simulink model "Laengsdynamikmodell_NEmo_MonteCarlo"  (R2019b)
settings: Solver=FixedStepAuto  StartTime=0.0  StopTime=1  FixedStep=SampleTime  RelTol=1e-3
undefined symbols (not defined in the file): C_RR, DiscIntNeverNeededParam, gravity, OM_PEl_M_Map, omega_Mot, PEl_MotVector, power_map_Mot, r_dyn, torque_Mot, UncertaintyMappedLosses, UncertaintyRollerDynamometer, UncertaintyTabledConsumption, VehMass
libraries: Driver_PI x1, Longitudinal_DrivingCycles x1, Acceleration_Calculation x1, Air_Resistance x1, Roll_Resistance x1, Slope_Resistance x1, Simple_Auxiliary x1, Gear_Stage x1, DCAC_Converter x1
(part 2 of 2)

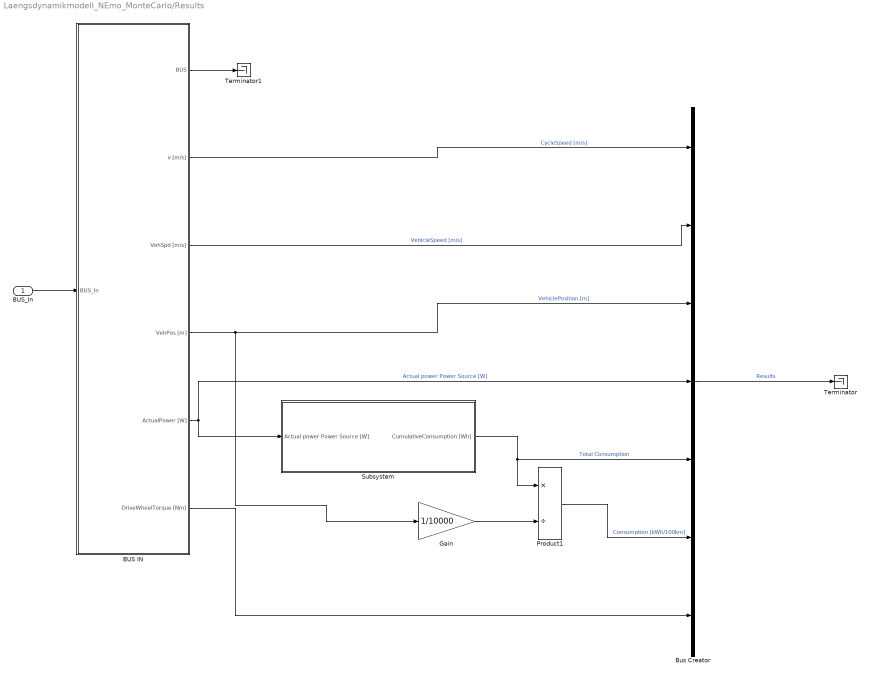
== system Laengsdynamikmodell_NEmo_MonteCarlo/Results ==
  BUS_In : Inport
  BUS IN : Subsystem
      mask help:
      | <Author> Alexander Koch
      | <Date> 02/05/2017
      | <Predecessor> Stefan Müller, Stephan Rohr
      |
      | <Description>
      | Automated BUS IN Block for the Bus System. After the Bus In is connected and receives signals it is possible to choose the required signals by clicking on the block. After choosing the signals it is possible to push the Refresh button. This button builds the required amount of outputs, connects the Bus Selector and the Outputs and rename all the outputs with the corresponding signal name.
      |
      | The Block automaticlly disconnects the link to the library block after opening the first time
      |
      | <Parameters>
      | -
      |
      | <Inputs>
      | Bus [Bus]
      |
      | <Outputs>
      | Bus [Bus]
      | SignalName[-]
      mask init:
      | BusInInitFct()
      settings: OpenFcn=|
      | set_param(gcb(),'LinkStatus','none')
      | open_system(gcb(),'mask')
      | open_system(strcat(gcb(),'/Bus Selector'),'Parameter')
      mask DialogControl ParameterGroupVar Prompt: Refresh
      mask DialogControl RefreshOutputs Prompt: Refresh all Output Names
      mask DialogControl RefreshOutputs Callback: BusInInitFct()
  Bus Creator : BusCreator  Inputs=7
  Gain : Gain  Gain=1/10000
  Product1 : Product  Inputs=*/
  Subsystem : Subsystem
  Terminator : Terminator
  Terminator1 : Terminator
  wires:
  BUS_In/1 -> BUS IN/1(BUS_In)
  BUS IN/1(BUS) -> Terminator1/1
  Bus Creator/1 -> Terminator/1  "Results"
  BUS IN/5(ActualPower [W]) -> Bus Creator/4, Subsystem/1(Actual power Power Source [W])  "Actual power Power Source [W]"
  BUS IN/2(v [m/s]) -> Bus Creator/1  "CycleSpeed [m/s]"
  BUS IN/3(VehSpd [m/s]) -> Bus Creator/2  "VehicleSpeed [m/s]"
  BUS IN/4(VehPos [m]) -> Bus Creator/3, Gain/1  "VehiclePosition [m]"
  BUS IN/6(DriveWheelTorque [Nm]) -> Bus Creator/7
  Gain/1 -> Product1/2
  Product1/1 -> Bus Creator/6  "Consumption [kWh/100km]"
  Subsystem/1(CumulativeConsumption [Wh]) -> Bus Creator/5, Product1/1  "Total Consumption"

== system Laengsdynamikmodell_NEmo_MonteCarlo/Timer and Bus Reset ==
  BUS_In : Inport
  Bus Creator : BusCreator  Inputs=1
  Bus Selector : BusSelector  OutputSignals=Dynamics,Powertrain,Powersource,VehicleControlUnit,Driver and Enironment,DrivinCycle  OutputAsBus=on
  Unit Delay : UnitDelay  SampleTime=-1  HasFrameUpgradeWarning=on
  BUS_Out : Outport  VectorParamsAs1DForOutWhenUnconnected=off
  wires:
  Bus Creator/1 -> BUS_Out/1
  Bus Selector/1 -> Unit Delay/1
  Unit Delay/1 -> Bus Creator/1  "Bus_Old"
  BUS_In/1 -> Bus Selector/1

== system Laengsdynamikmodell_NEmo_MonteCarlo/Vehicle Control Unit ==
  BUS_In : Inport
  BUS IN : Subsystem
      mask help:
      | <Author> Alexander Koch based on Stefan Müller, Stephan Rohr
      | <Date> 02/05/2017
      |
      | <Description>
      | Automated BUS IN Block for the Bus System. After the Bus In is connected and receives signals it is possible to choose the required signals by clicking on the block. After choosing the signals it is possible to push the Refresh button. This button builds the required amount of outputs, connects the Bus Selector and the Outputs and rename all the outputs with the corresponding signal name.
      |
      | The Block automaticlly disconnects the link to the library block after opening the first time
      |
      | <Parameters>
      | -
      |
      | <Inputs>
      | Bus [Bus]
      |
      | <Outputs>
      | Bus [Bus]
      | SignalName[-]
      mask init:
      | BusInInitFct()
      settings: OpenFcn=|
      | set_param(gcb(),'LinkStatus','none')
      | open_system(gcb(),'mask')
      | open_system(strcat(gcb(),'/Bus Selector'),'Parameter')
      mask DialogControl ParameterGroupVar Prompt: Refresh
      mask DialogControl RefreshOutputs Prompt: Refresh all Output Names
      mask DialogControl RefreshOutputs Callback: BusInInitFct()
  BUS OUT : Subsystem  mask{NumberofInputs=3, NameSys='VehicleControlUnit'}
      mask prompts: NumberofInputs "Numper of costum inputs"; NameSys "Name of Bus Subsystem"
      mask help:
      | <Author> Alexander Koch based on Stefan Müller, Stephan Rohr
      | <Date> 02/05/2017
      |
      | <Description>
      | Automated BUS Out Block for the Bus System. Allows to enter the Number of costum inputs and the name of the bus system. After entering the parameters the required amout of Inputs are built and connected to the Bus Creator. The signal names that are connected to the inputs In1, ..., InN are automatically adopted at the Bus signal names and can be found in the Bus under the name of the Bus Subsystem. If the signal (line) to the Inport has no name, the name of the previous blocks outport is taken. If this is not possible, the name if the previous block is taken for the Bus signal name.
      |
      | Additional, there are two buttons. The Refresh Input Names refreshes all Input Names. This is required if signal names are changed or signals are connected for the first time. To build a new system or if another Subsystem is added between existing subsystems, the Refresh Bus Selector is required at every subsystem that is calculated after the new subsystem.
      |
      | The Block automaticlly disconnects the link to the library block after opening the first time
      |
      | <Parameters>
      | Number of costum inputs [-]
      | Name of Bus Subsystem ['abc']
      |
      | <Inputs>
      | Bus [Bus]
      | In1 [ ]
      |
      | <Outputs>
      | Bus [Bus]
      mask init:
      | BusRefreshInputs()
      settings: OpenFcn=|
      | set_param(gcb(),'LinkStatus','none')
      | open_system(gcb(),'mask')
      mask DialogControl Container3 Prompt: Refresh
      mask DialogControl RefreshInputNames Prompt: Refresh Input Names
      mask DialogControl RefreshInputNames Callback: BusRefreshLineNames()
      mask DialogControl RefreshBusSelector Prompt: Refresh Bus Selector
      mask DialogControl RefreshBusSelector Callback: BusRefreshBusSelector()
  Control Unit Simple : Subsystem  AncestorBlock=Control_Unit_Simple/Control Unit Simple  mask(SB){Brake_Distribution_Front=0.7, MaxBrkTrq=448, MaxMotorTrq=110}
      mask prompts: Brake_Distribution_Front "Brake Distribution Front"; MaxBrkTrq "Maximal Braking Torque"; MaxMotorTrq "Maximal Motor Torque"
      mask help:
      | <Author> Alexander Koch based on Stefan Müller, Stephan Rohr </Author>
      | <Date> 03/04/2017 </Date>
      |
      | <Description>
      | Requires acceleration pedal position, braking pedal position, a brake distribution, the maximal possible braking torque and tha maximal motor torque and calculates a target drive system torque and a target braking torque for front and rear axle. Minimum drive torques is zero.
      | </Description>
      mask Help:
      | <Parameters>
      | Brake distribution front [-]
      | 	<Min> 0 </Min>
      | 	<Max> 1 </Max>
      | Maximal braking torque [Nm]
      | Maximal motor torque [Nm]
      | </Parameters>
      | 
      | <Inputs>
      | AccPedalPos [-]
      | 	<Min> 0 </Min>
      | 	<Max> 1 </Max>
      | BrakePedalPos [-]
      | 	<Min>0 </Min>
      | 	<Max> 1 </Max>
      | </Inputs>
      | 
      | <Outputs>
      | TargetDriveTrq [Nm]
      | 	<Min> 0 </Min>
      | TargetBrakeTrqFrontAxle [Nm]
      | 	<Max> 0 </Max>
      | TargetBrakeTrqRearAxle [Nm]
      | 	<Max> 0 </Max>
      | </Outputs>
      mask TypeOptions Brake_Distribution_Front: Brake_Distribution_Front/Value
      mask TypeOptions MaxBrkTrq: MaxBrakeTorque/Value
      mask TypeOptions MaxMotorTrq: MaxMotorTorque/Value
      mask DialogControl Container3 Prompt: Documentation:
      mask DialogControl DescHelpVar Prompt: %<MaskHelp>
  BUS_Out : Outport  VectorParamsAs1DForOutWhenUnconnected=off
  wires:
  BUS IN/1(BUS) -> BUS OUT/1(BUS)
  BUS OUT/1(BUS_OUT) -> BUS_Out/1
  BUS_In/1 -> BUS IN/1(BUS_In)
  Control Unit Simple/2(TargetBrakeTrqFrontAxle [Nm]) -> BUS OUT/3(In2)
  Control Unit Simple/3(TargetBrakeTrqRearAxle [Nm]) -> BUS OUT/4(In3)
  Control Unit Simple/1("TargetDriveTrq [Nm] ") -> BUS OUT/2(In1)
  BUS IN/2(AccPedalPos [-]) -> Control Unit Simple/1(AccPedalPos [-])
  BUS IN/3(BrakePedalPos [-]) -> Control Unit Simple/2(BrakePedalPos [-])

== system Laengsdynamikmodell_NEmo_MonteCarlo/Driver and Environment/BUS IN ==
  BUS_In : Inport
  Bus Selector : BusSelector  OutputSignals=DrivinCycle.v [m/s],Bus_Old.Dynamics.VehSpd [m/s]
  BUS : Outport  VectorParamsAs1DForOutWhenUnconnected=off
  v [m/s] : Outport  Port=2  VectorParamsAs1DForOutWhenUnconnected=off
  VehSpd [m/s] : Outport  Port=3  VectorParamsAs1DForOutWhenUnconnected=off
  wires:
  BUS_In/1 -> Bus Selector/1, BUS/1
  Bus Selector/1 -> v [m/s]/1  "<v [m/s]>"
  Bus Selector/2 -> VehSpd [m/s]/1  "<VehSpd [m/s]>"

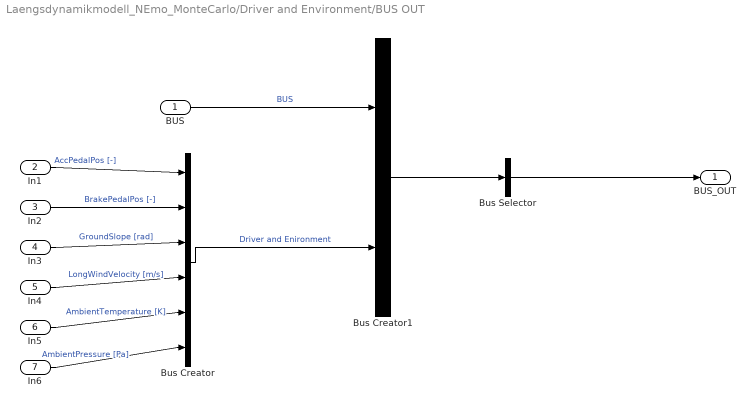
== system Laengsdynamikmodell_NEmo_MonteCarlo/Driver and Environment/BUS OUT ==
  BUS : Inport
  In1 : Inport  Port=2
  In2 : Inport  Port=3
  In3 : Inport  Port=4
  In4 : Inport  Port=5
  In5 : Inport  Port=6
  In6 : Inport  Port=7
  Bus Creator : BusCreator  Inputs=NumberofInputs
  Bus Creator1 : BusCreator  Inputs=2
  Bus Selector : BusSelector  OutputSignals=Driver and Enironment,BUS.DrivinCycle,BUS.Bus_Old  OutputAsBus=on
  BUS_OUT : Outport  VectorParamsAs1DForOutWhenUnconnected=off
  wires:
  Bus Creator1/1 -> Bus Selector/1
  BUS/1 -> Bus Creator1/1  "BUS"
  Bus Creator/1 -> Bus Creator1/2  "Driver and Enironment"
  Bus Selector/1 -> BUS_OUT/1
  In1/1 -> Bus Creator/1  "AccPedalPos [-]"
  In2/1 -> Bus Creator/2  "BrakePedalPos [-]"
  In3/1 -> Bus Creator/3  "GroundSlope [rad]"
  In4/1 -> Bus Creator/4  "LongWindVelocity [m/s]"
  In5/1 -> Bus Creator/5  "AmbientTemperature [K]"
  In6/1 -> Bus Creator/6  "AmbientPressure [Pa]"

== system Laengsdynamikmodell_NEmo_MonteCarlo/Driver and Environment/Constant Environment ==
  Const_Ambient_Pressure : Constant  Value=Ambient_P  SampleTime=LocalSampleTime
  Const_Ambient_Temperature : Constant  Value=Ambient_Temp  SampleTime=LocalSampleTime
  Const_Ground_Slope : Constant  Value=Ground_Slope  SampleTime=LocalSampleTime
  Const_Long_Wind_Velocity : Constant  Value=Long_Wind_Speed  SampleTime=LocalSampleTime
  GroundSlope [rad] : Outport  SampleTime=GlobalSampleTime  VectorParamsAs1DForOutWhenUnconnected=off
  LongWindVelocity [m/s] : Outport  Port=2  SampleTime=GlobalSampleTime  VectorParamsAs1DForOutWhenUnconnected=off
  AmbientTemperature [K] : Outport  Port=3  SampleTime=GlobalSampleTime  VectorParamsAs1DForOutWhenUnconnected=off
  AmbientPressure [Pa] : Outport  Port=4  SampleTime=GlobalSampleTime  VectorParamsAs1DForOutWhenUnconnected=off
  wires:
  Const_Ambient_Pressure/1 -> AmbientPressure [Pa]/1
  Const_Ambient_Temperature/1 -> AmbientTemperature [K]/1
  Const_Ground_Slope/1 -> GroundSlope [rad]/1
  Const_Long_Wind_Velocity/1 -> LongWindVelocity [m/s]/1

== system Laengsdynamikmodell_NEmo_MonteCarlo/Driving Cycle/BUS IN ==
  BUS_In : Inport
  Bus Selector : BusSelector  OutputSignals=Bus_Old.Dynamics.VehSpd [m/s]
  BUS : Outport  VectorParamsAs1DForOutWhenUnconnected=off
  VehSpd [m/s] : Outport  Port=2  VectorParamsAs1DForOutWhenUnconnected=off
  wires:
  BUS_In/1 -> Bus Selector/1, BUS/1
  Bus Selector/1 -> VehSpd [m/s]/1  "<VehSpd [m/s]>"

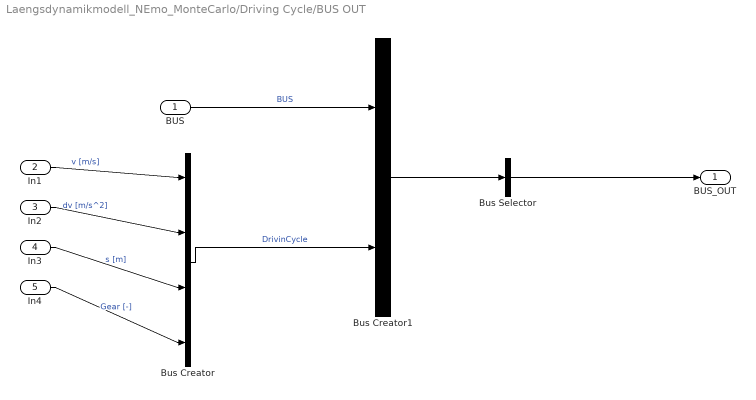
== system Laengsdynamikmodell_NEmo_MonteCarlo/Driving Cycle/BUS OUT ==
  BUS : Inport
  In1 : Inport  Port=2
  In2 : Inport  Port=3
  In3 : Inport  Port=4
  In4 : Inport  Port=5
  Bus Creator : BusCreator  Inputs=NumberofInputs
  Bus Creator1 : BusCreator  Inputs=2
  Bus Selector : BusSelector  OutputSignals=DrivinCycle,BUS.Bus_Old  OutputAsBus=on
  BUS_OUT : Outport  VectorParamsAs1DForOutWhenUnconnected=off
  wires:
  Bus Creator1/1 -> Bus Selector/1
  BUS/1 -> Bus Creator1/1  "BUS"
  Bus Creator/1 -> Bus Creator1/2  "DrivinCycle"
  Bus Selector/1 -> BUS_OUT/1
  In1/1 -> Bus Creator/1  "v [m/s]"
  In2/1 -> Bus Creator/2  "dv [m/s^2]"
  In3/1 -> Bus Creator/3  "s [m]"
  In4/1 -> Bus Creator/4  "Gear [-]"

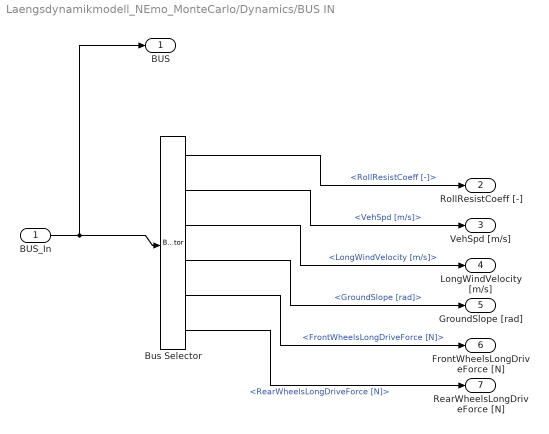
== system Laengsdynamikmodell_NEmo_MonteCarlo/Dynamics/BUS IN ==
  BUS_In : Inport
  Bus Selector : BusSelector  OutputSignals=Powertrain.RollResistCoeff [-],Bus_Old.Dynamics.VehSpd [m/s],Driver and Enironment.LongWindVelocity [m/s],Driver and Enironment.GroundSlope [rad],Powertrain.FrontWheelsLongDriveForce [N],Powertrain.RearWheelsLongDriveForce [N]
  BUS : Outport  VectorParamsAs1DForOutWhenUnconnected=off
  RollResistCoeff [-] : Outport  Port=2  VectorParamsAs1DForOutWhenUnconnected=off
  VehSpd [m/s] : Outport  Port=3  VectorParamsAs1DForOutWhenUnconnected=off
  LongWindVelocity [m/s] : Outport  Port=4  VectorParamsAs1DForOutWhenUnconnected=off
  GroundSlope [rad] : Outport  Port=5  VectorParamsAs1DForOutWhenUnconnected=off
  FrontWheelsLongDriveForce [N] : Outport  Port=6  VectorParamsAs1DForOutWhenUnconnected=off
  RearWheelsLongDriveForce [N] : Outport  Port=7  VectorParamsAs1DForOutWhenUnconnected=off
  wires:
  BUS_In/1 -> Bus Selector/1, BUS/1
  Bus Selector/1 -> RollResistCoeff [-]/1  "<RollResistCoeff [-]>"
  Bus Selector/2 -> VehSpd [m/s]/1  "<VehSpd [m/s]>"
  Bus Selector/3 -> LongWindVelocity [m/s]/1  "<LongWindVelocity [m/s]>"
  Bus Selector/4 -> GroundSlope [rad]/1  "<GroundSlope [rad]>"
  Bus Selector/5 -> FrontWheelsLongDriveForce [N]/1  "<FrontWheelsLongDriveForce [N]>"
  Bus Selector/6 -> RearWheelsLongDriveForce [N]/1  "<RearWheelsLongDriveForce [N]>"

== system Laengsdynamikmodell_NEmo_MonteCarlo/Dynamics/BUS OUT ==
  BUS : Inport
  In1 : Inport  Port=2
  In2 : Inport  Port=3
  In3 : Inport  Port=4
  Bus Creator : BusCreator  Inputs=NumberofInputs
  Bus Creator1 : BusCreator  Inputs=2
  Bus Selector : BusSelector  OutputSignals=Dynamics,BUS.Powertrain,BUS.Powersource,BUS.VehicleControlUnit,BUS.Driver and Enironment,BUS.DrivinCycle,BUS.Bus_Old  OutputAsBus=on
  BUS_OUT : Outport  VectorParamsAs1DForOutWhenUnconnected=off
  wires:
  Bus Creator1/1 -> Bus Selector/1
  BUS/1 -> Bus Creator1/1  "BUS"
  Bus Creator/1 -> Bus Creator1/2  "Dynamics"
  Bus Selector/1 -> BUS_OUT/1
  In1/1 -> Bus Creator/1  "Acc [m/s^2]"
  In2/1 -> Bus Creator/2  "VehSpd [m/s]"
  In3/1 -> Bus Creator/3  "VehPos [m]"

== system Laengsdynamikmodell_NEmo_MonteCarlo/Power Source/BUS IN ==
  BUS_In : Inport
  Bus Selector : BusSelector  OutputSignals=Bus_Old.Powertrain.PowertrainPowerReq [W]
  BUS : Outport  VectorParamsAs1DForOutWhenUnconnected=off
  PowertrainPowerReq [W] : Outport  Port=2  VectorParamsAs1DForOutWhenUnconnected=off
  wires:
  BUS_In/1 -> Bus Selector/1, BUS/1
  Bus Selector/1 -> PowertrainPowerReq [W]/1  "<PowertrainPowerReq [W]>"

== system Laengsdynamikmodell_NEmo_MonteCarlo/Power Source/BUS OUT ==
  BUS : Inport
  In1 : Inport  Port=2
  In2 : Inport  Port=3
  In3 : Inport  Port=4
  Bus Creator : BusCreator  Inputs=NumberofInputs
  Bus Creator1 : BusCreator  Inputs=2
  Bus Selector : BusSelector  OutputSignals=Powersource,BUS.VehicleControlUnit,BUS.Driver and Enironment,BUS.DrivinCycle,BUS.Bus_Old  OutputAsBus=on
  BUS_OUT : Outport  VectorParamsAs1DForOutWhenUnconnected=off
  wires:
  Bus Creator1/1 -> Bus Selector/1
  BUS/1 -> Bus Creator1/1  "BUS"
  Bus Creator/1 -> Bus Creator1/2  "Powersource"
  Bus Selector/1 -> BUS_OUT/1
  In1/1 -> Bus Creator/1  "ActualPower [W]"
  In2/1 -> Bus Creator/2  "MaxPower [W]"
  In3/1 -> Bus Creator/3  "MinPower [W]"

== system Laengsdynamikmodell_NEmo_MonteCarlo/Power Source/Constant Power Source ==
  RequiredPower [W] : Inport
  Constant : Constant  Value=MaxPower
  Constant1 : Constant  Value=MinPower
  Saturation : Saturate  UpperLimit=MaxPower  LowerLimit=MinPower
  ActualPower [W] : Outport  VectorParamsAs1DForOutWhenUnconnected=off
  MaxPower [W] : Outport  Port=2  VectorParamsAs1DForOutWhenUnconnected=off
  MinPower [W] : Outport  Port=3  VectorParamsAs1DForOutWhenUnconnected=off
  wires:
  Constant/1 -> MaxPower [W]/1
  Constant1/1 -> MinPower [W]/1
  Saturation/1 -> ActualPower [W]/1
  RequiredPower [W]/1 -> Saturation/1

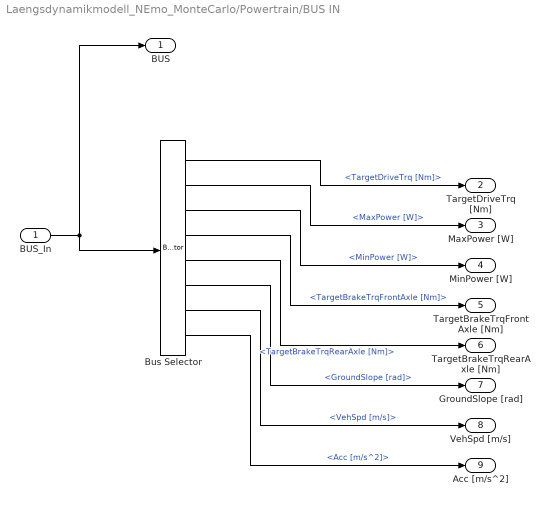
== system Laengsdynamikmodell_NEmo_MonteCarlo/Powertrain/BUS IN ==
  BUS_In : Inport
  Bus Selector : BusSelector  OutputSignals=VehicleControlUnit.TargetDriveTrq [Nm],Powersource.MaxPower [W],Powersource.MinPower [W],VehicleControlUnit.TargetBrakeTrqFrontAxle [Nm],VehicleControlUnit.TargetBrakeTrqRearAxle [Nm],Driver and Enironment.GroundSlope [rad],Bus_Old.Dynamics.VehSpd [m/s],Bus_Old.Dynamics.Acc [m/s^2]
  BUS : Outport  VectorParamsAs1DForOutWhenUnconnected=off
  TargetDriveTrq [Nm] : Outport  Port=2  VectorParamsAs1DForOutWhenUnconnected=off
  MaxPower [W] : Outport  Port=3  VectorParamsAs1DForOutWhenUnconnected=off
  MinPower [W] : Outport  Port=4  VectorParamsAs1DForOutWhenUnconnected=off
  TargetBrakeTrqFrontAxle [Nm] : Outport  Port=5  VectorParamsAs1DForOutWhenUnconnected=off
  TargetBrakeTrqRearAxle [Nm] : Outport  Port=6  VectorParamsAs1DForOutWhenUnconnected=off
  GroundSlope [rad] : Outport  Port=7  VectorParamsAs1DForOutWhenUnconnected=off
  VehSpd [m/s] : Outport  Port=8  VectorParamsAs1DForOutWhenUnconnected=off
  Acc [m/s^2] : Outport  Port=9  VectorParamsAs1DForOutWhenUnconnected=off
  wires:
  BUS_In/1 -> Bus Selector/1, BUS/1
  Bus Selector/1 -> TargetDriveTrq [Nm]/1  "<TargetDriveTrq [Nm]>"
  Bus Selector/2 -> MaxPower [W]/1  "<MaxPower [W]>"
  Bus Selector/3 -> MinPower [W]/1  "<MinPower [W]>"
  Bus Selector/4 -> TargetBrakeTrqFrontAxle [Nm]/1  "<TargetBrakeTrqFrontAxle [Nm]>"
  Bus Selector/5 -> TargetBrakeTrqRearAxle [Nm]/1  "<TargetBrakeTrqRearAxle [Nm]>"
  Bus Selector/6 -> GroundSlope [rad]/1  "<GroundSlope [rad]>"
  Bus Selector/7 -> VehSpd [m/s]/1  "<VehSpd [m/s]>"
  Bus Selector/8 -> Acc [m/s^2]/1  "<Acc [m/s^2]>"

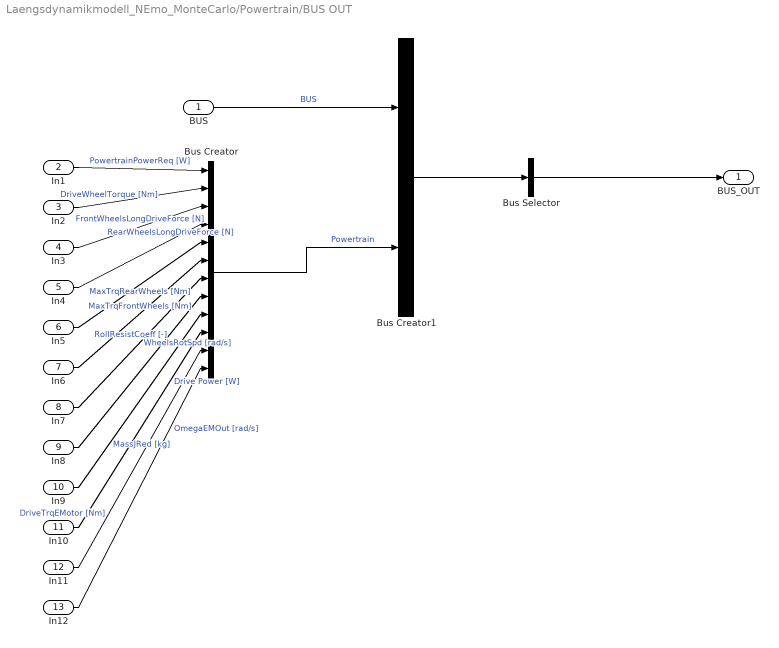
== system Laengsdynamikmodell_NEmo_MonteCarlo/Powertrain/BUS OUT ==
  BUS : Inport
  In1 : Inport  Port=2
  In2 : Inport  Port=3
  In3 : Inport  Port=4
  In4 : Inport  Port=5
  In5 : Inport  Port=6
  In6 : Inport  Port=7
  In7 : Inport  Port=8
  In8 : Inport  Port=9
  In9 : Inport  Port=10
  In10 : Inport  Port=11
  In11 : Inport  Port=12
  In12 : Inport  Port=13
  Bus Creator : BusCreator  Inputs=NumberofInputs
  Bus Creator1 : BusCreator  Inputs=2
  Bus Selector : BusSelector  OutputSignals=Powertrain,BUS.Powersource,BUS.VehicleControlUnit,BUS.Driver and Enironment,BUS.DrivinCycle,BUS.Bus_Old  OutputAsBus=on
  BUS_OUT : Outport  VectorParamsAs1DForOutWhenUnconnected=off
  wires:
  Bus Creator1/1 -> Bus Selector/1
  BUS/1 -> Bus Creator1/1  "BUS"
  Bus Creator/1 -> Bus Creator1/2  "Powertrain"
  Bus Selector/1 -> BUS_OUT/1
  In1/1 -> Bus Creator/1  "PowertrainPowerReq [W]"
  In2/1 -> Bus Creator/2  "DriveWheelTorque [Nm]"
  In3/1 -> Bus Creator/3  "FrontWheelsLongDriveForce [N]"
  In4/1 -> Bus Creator/4  "RearWheelsLongDriveForce [N]"
  In5/1 -> Bus Creator/5  "MaxTrqRearWheels [Nm]"
  In6/1 -> Bus Creator/6  "MaxTrqFrontWheels [Nm]"
  In7/1 -> Bus Creator/7  "WheelsRotSpd [rad/s]"
  In8/1 -> Bus Creator/8  "RollResistCoeff [-]"
  In9/1 -> Bus Creator/9  "MassJRed [kg]"
  In10/1 -> Bus Creator/10  "Drive Power [W]"
  In11/1 -> Bus Creator/11  "DriveTrqEMotor [Nm]"
  In12/1 -> Bus Creator/12  "OmegaEMOut [rad/s]"

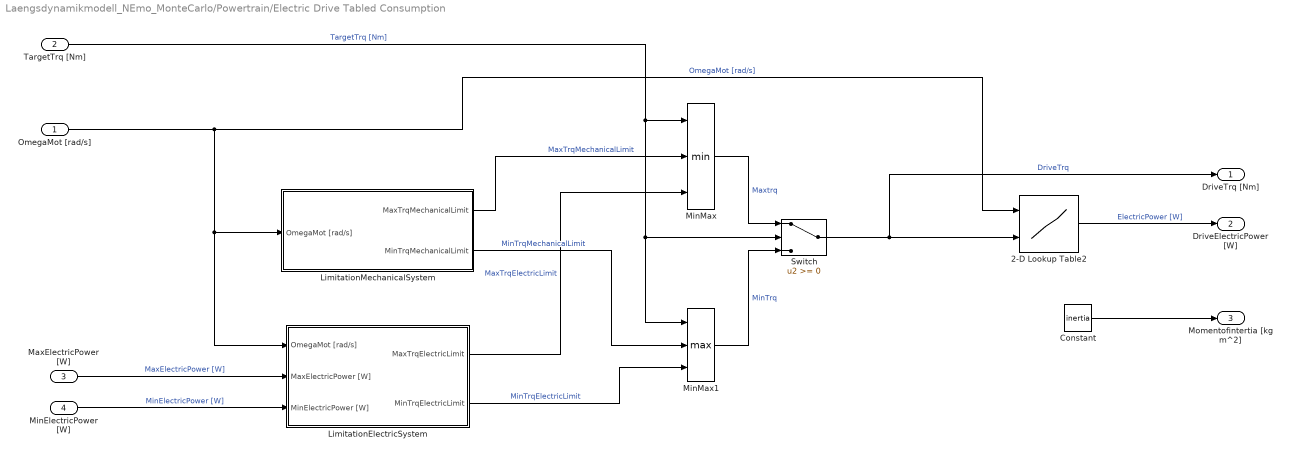
== system Laengsdynamikmodell_NEmo_MonteCarlo/Powertrain/Electric Drive Tabled Consumption ==
  OmegaMot [rad/s] : Inport  SampleTime=LocalSampleTime
  TargetTrq [Nm] : Inport  Port=2  SampleTime=LocalSampleTime
  MaxElectricPower [W] : Inport  Port=3  SampleTime=LocalSampleTime
  MinElectricPower [W] : Inport  Port=4  SampleTime=LocalSampleTime
  2-D Lookup Table2 : Lookup_n-D  BreakpointsForDimension1=OM_MotVector  BreakpointsForDimension2=M_MotVector  Table=OM_M_Pel_Map  UseLastTableValue=on  InternalRulePriority=Speed  RndMeth=Simplest  InputSameDT=on
  Constant : Constant  Value=inertia
  LimitationElectricSystem : Subsystem
  LimitationMechanicalSystem : Subsystem
  MinMax : MinMax  Inputs=3
  MinMax1 : MinMax  Function=max  Inputs=3
  Switch : Switch
  DriveTrq [Nm] : Outport  SampleTime=GlobalSampleTime  VectorParamsAs1DForOutWhenUnconnected=off
  DriveElectricPower [W] : Outport  Port=2  SampleTime=GlobalSampleTime  VectorParamsAs1DForOutWhenUnconnected=off
  Momentofintertia [kg m^2] : Outport  Port=3  SampleTime=GlobalSampleTime  VectorParamsAs1DForOutWhenUnconnected=off
  wires:
  Constant/1 -> Momentofintertia [kg m^2]/1
  LimitationElectricSystem/1(MaxTrqElectricLimit) -> MinMax/3  "MaxTrqElectricLimit"
  LimitationElectricSystem/2(MinTrqElectricLimit) -> MinMax1/3  "MinTrqElectricLimit"
  LimitationMechanicalSystem/2(MinTrqMechanicalLimit) -> MinMax1/2  "MinTrqMechanicalLimit"
  LimitationMechanicalSystem/1(MaxTrqMechanicalLimit) -> MinMax/2  "MaxTrqMechanicalLimit"
  MinElectricPower [W]/1 -> LimitationElectricSystem/3(MinElectricPower [W])  "MinElectricPower [W]"
  MaxElectricPower [W]/1 -> LimitationElectricSystem/2(MaxElectricPower [W])  "MaxElectricPower [W]"
  OmegaMot [rad/s]/1 -> 2-D Lookup Table2/1, LimitationMechanicalSystem/1(OmegaMot [rad/s]), LimitationElectricSystem/1(OmegaMot [rad/s])  "OmegaMot [rad/s]"
  Switch/1 -> DriveTrq [Nm]/1, 2-D Lookup Table2/2  "DriveTrq"
  TargetTrq [Nm]/1 -> MinMax/1, Switch/2, MinMax1/1  "TargetTrq [Nm]"
  MinMax1/1 -> Switch/3  "MinTrq"
  MinMax/1 -> Switch/1  "Maxtrq"
  2-D Lookup Table2/1 -> DriveElectricPower [W]/1  "ElectricPower [W]"

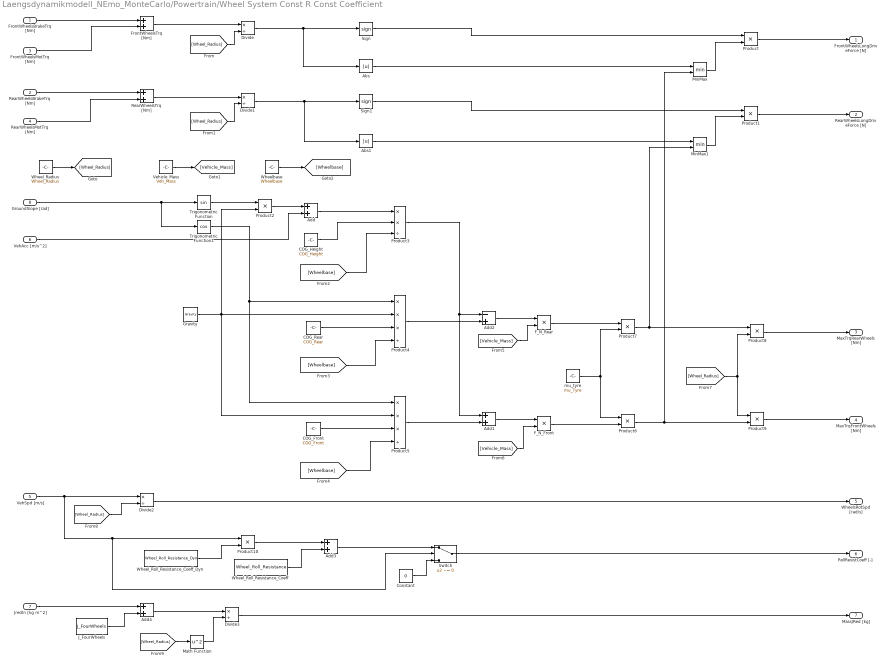
== system Laengsdynamikmodell_NEmo_MonteCarlo/Powertrain/Wheel System Const R Const Coefficient ==
  FrontWheelsBrakeTrq [Nm] : Inport  SampleTime=LocalSampleTime
  RearWheelsBrakeTrq [Nm] : Inport  Port=2  SampleTime=LocalSampleTime
  FrontWheelsMotTrq [Nm] : Inport  Port=3  SampleTime=LocalSampleTime
  RearWheelsMotTrq [Nm] : Inport  Port=4  SampleTime=LocalSampleTime
  VehSpd [m/s] : Inport  Port=5  SampleTime=LocalSampleTime
  VehAcc [m/s^2] : Inport  Port=6  SampleTime=LocalSampleTime
  JredIn [kg m^2] : Inport  Port=7  SampleTime=LocalSampleTime
  GroundSlope [rad] : Inport  Port=8  SampleTime=LocalSampleTime
  Abs : Abs
  Abs1 : Abs
  Add{,1,3..4} (4 alike) : Sum
  Add2 : Sum  Inputs=-+
  COG_Front : Constant  Value=COG_Front
  COG_Height : Constant  Value=COG_Height
  COG_Rear : Constant  Value=COG_Rear
  Constant : Constant  Value=0
  Divide{,1..3} (4 alike) : Product  Inputs=*/
  F_N_Front : Product
  F_N_Rear : Product
  FrontWheelsTrq [Nm] : Sum
  Gravity : Constant  Value=Gravity
  J_FourWheels : Constant  Value=J_FourWheels
  Math Function : Math  Operator=square  SaturateOnIntegerOverflow=on
  MinMax : MinMax  Inputs=2
  MinMax1 : MinMax  Inputs=2
  Product{,1..2,6..10} (8 alike) : Product
  Product3 : Product  Inputs=**/
  Product4 : Product  Inputs=***/
  Product5 : Product  Inputs=***/
  RearWheelsTrq [Nm] : Sum
  Sign : Signum
  Sign1 : Signum
  Switch : Switch  Criteria=u2 ~= 0
  Trigonometric Function : Trigonometry
  Trigonometric Function1 : Trigonometry  Operator=cos
  Vehicle_Mass : Constant  Value=Veh_Mass
  Wheel_Radius : Constant  Value=Wheel_Radius
  Wheel_Roll_Resistance_Coeff : Constant  Value=Wheel_Roll_Resistance
  Wheel_Roll_Resistance_Coeff_Dyn : Constant  Value=Wheel_Roll_Resistance_Dyn
  Wheelbase : Constant  Value=Wheelbase
  mu_tyre : Constant  Value=mu_Tyre
  FrontWheelsLongDriveForce [N] : Outport  SampleTime=GlobalSampleTime  VectorParamsAs1DForOutWhenUnconnected=off
  RearWheelsLongDriveForce [N] : Outport  Port=2  SampleTime=GlobalSampleTime  VectorParamsAs1DForOutWhenUnconnected=off
  MaxTrqRearWheels [Nm] : Outport  Port=3  SampleTime=GlobalSampleTime  VectorParamsAs1DForOutWhenUnconnected=off
  MaxTrqFrontWheels [Nm] : Outport  Port=4  SampleTime=GlobalSampleTime  VectorParamsAs1DForOutWhenUnconnected=off
  WheelsRotSpd [rad/s] : Outport  Port=5  SampleTime=GlobalSampleTime  VectorParamsAs1DForOutWhenUnconnected=off
  RollResistCoeff [-] : Outport  Port=6  SampleTime=GlobalSampleTime  VectorParamsAs1DForOutWhenUnconnected=off
  MassJRed [kg] : Outport  Port=7  SampleTime=GlobalSampleTime  VectorParamsAs1DForOutWhenUnconnected=off
  wires:
  Divide3/1 -> MassJRed [kg]/1
  [Wheel_Radius] -> Math Function/1
  Math Function/1 -> Divide3/2
  Add4/1 -> Divide3/1
  J_FourWheels/1 -> Add4/2
  JredIn [kg m^2]/1 -> Add4/1
  Switch/1 -> RollResistCoeff [-]/1
  Constant/1 -> Switch/3
  Add3/1 -> Switch/1
  Wheel_Roll_Resistance_Coeff/1 -> Add3/2
  Product10/1 -> Add3/1
  Wheel_Roll_Resistance_Coeff_Dyn/1 -> Product10/2
  Divide2/1 -> WheelsRotSpd [rad/s]/1
  [Wheel_Radius] -> Divide2/2
  VehSpd [m/s]/1 -> Divide2/1, Product10/1, Switch/2
  Product9/1 -> MaxTrqFrontWheels [Nm]/1
  Product8/1 -> MaxTrqRearWheels [Nm]/1
  [Wheel_Radius] -> Product9/1, Product8/2
  Product7/1 -> MinMax1/2, Product8/1
  Product6/1 -> MinMax/2, Product9/2
  mu_tyre/1 -> Product7/2, Product6/1
  F_N_Front/1 -> Product6/2
  F_N_Rear/1 -> Product7/1
  [Vehicle_Mass] -> F_N_Front/2
  [Vehicle_Mass] -> F_N_Rear/2
  Add1/1 -> F_N_Front/1
  Add2/1 -> F_N_Rear/1
  Product4/1 -> Add2/2
  Product3/1 -> Add1/1, Add2/1
  Product5/1 -> Add1/2
  [Wheelbase] -> Product5/4
  COG_Front/1 -> Product5/3
  [Wheelbase] -> Product4/4
  [Wheelbase] -> Product3/3
  Wheelbase/1 -> [Wheelbase]
  COG_Rear/1 -> Product4/3
  Gravity/1 -> Product4/2, Product5/2, Product2/2
  Trigonometric Function1/1 -> Product5/1, Product4/1
  COG_Height/1 -> Product3/2
  Add/1 -> Product3/1
  VehAcc [m/s^2]/1 -> Add/2
  Product2/1 -> Add/1
  Trigonometric Function/1 -> Product2/1
  GroundSlope [rad]/1 -> Trigonometric Function/1, Trigonometric Function1/1
  Vehicle_Mass/1 -> [Vehicle_Mass]
  Product1/1 -> RearWheelsLongDriveForce [N]/1
  MinMax1/1 -> Product1/2
  Sign1/1 -> Product1/1
  Abs1/1 -> MinMax1/1
  Divide1/1 -> Sign1/1, Abs1/1
  [Wheel_Radius] -> Divide1/2
  [Wheel_Radius] -> Divide/2
  Wheel_Radius/1 -> [Wheel_Radius]
  MinMax/1 -> Product/2
  Abs/1 -> MinMax/1
  Divide/1 -> Sign/1, Abs/1
  Sign/1 -> Product/1
  Product/1 -> FrontWheelsLongDriveForce [N]/1
  RearWheelsTrq [Nm]/1 -> Divide1/1
  FrontWheelsTrq [Nm]/1 -> Divide/1
  RearWheelsMotTrq [Nm]/1 -> RearWheelsTrq [Nm]/2
  RearWheelsBrakeTrq [Nm]/1 -> RearWheelsTrq [Nm]/1
  FrontWheelsMotTrq [Nm]/1 -> FrontWheelsTrq [Nm]/2
  FrontWheelsBrakeTrq [Nm]/1 -> FrontWheelsTrq [Nm]/1

== system Laengsdynamikmodell_NEmo_MonteCarlo/Results/BUS IN ==
  BUS_In : Inport
  Bus Selector : BusSelector  OutputSignals=DrivinCycle.v [m/s],Dynamics.VehSpd [m/s],Dynamics.VehPos [m],Powersource.ActualPower [W],Powertrain.DriveWheelTorque [Nm]
  BUS : Outport  VectorParamsAs1DForOutWhenUnconnected=off
  v [m/s] : Outport  Port=2  VectorParamsAs1DForOutWhenUnconnected=off
  VehSpd [m/s] : Outport  Port=3  VectorParamsAs1DForOutWhenUnconnected=off
  VehPos [m] : Outport  Port=4  VectorParamsAs1DForOutWhenUnconnected=off
  ActualPower [W] : Outport  Port=5  VectorParamsAs1DForOutWhenUnconnected=off
  DriveWheelTorque [Nm] : Outport  Port=6  VectorParamsAs1DForOutWhenUnconnected=off
  wires:
  BUS_In/1 -> BUS/1, Bus Selector/1
  Bus Selector/1 -> v [m/s]/1  "<v [m/s]>"
  Bus Selector/2 -> VehSpd [m/s]/1  "<VehSpd [m/s]>"
  Bus Selector/3 -> VehPos [m]/1  "<VehPos [m]>"
  Bus Selector/4 -> ActualPower [W]/1  "<ActualPower [W]>"
  Bus Selector/5 -> DriveWheelTorque [Nm]/1  "<DriveWheelTorque [Nm]>"

== system Laengsdynamikmodell_NEmo_MonteCarlo/Results/Subsystem ==
  Actual power Power Source [W] : Inport
  Discrete-Time Integrator : DiscreteIntegrator  SampleTime=-1  ICPrevOutput=DiscIntNeverNeededParam  ICPrevScaledInput=DiscIntNeverNeededParam
  Gain1 : Gain  Gain=1/3600
  CumulativeConsumption [Wh] : Outport  Unit=W*h
  wires:
  Discrete-Time Integrator/1 -> Gain1/1
  Gain1/1 -> CumulativeConsumption [Wh]/1  "CumulativeConsumption [Wh]"
  Actual power Power Source [W]/1 -> Discrete-Time Integrator/1

== system Laengsdynamikmodell_NEmo_MonteCarlo/Vehicle Control Unit/BUS IN ==
  BUS_In : Inport
  Bus Selector : BusSelector  OutputSignals=Driver and Enironment.AccPedalPos [-],Driver and Enironment.BrakePedalPos [-]
  BUS : Outport  VectorParamsAs1DForOutWhenUnconnected=off
  AccPedalPos [-] : Outport  Port=2  VectorParamsAs1DForOutWhenUnconnected=off
  BrakePedalPos [-] : Outport  Port=3  VectorParamsAs1DForOutWhenUnconnected=off
  wires:
  BUS_In/1 -> Bus Selector/1, BUS/1
  Bus Selector/1 -> AccPedalPos [-]/1  "<AccPedalPos [-]>"
  Bus Selector/2 -> BrakePedalPos [-]/1  "<BrakePedalPos [-]>"

== system Laengsdynamikmodell_NEmo_MonteCarlo/Vehicle Control Unit/BUS OUT ==
  BUS : Inport
  In1 : Inport  Port=2
  In2 : Inport  Port=3
  In3 : Inport  Port=4
  Bus Creator : BusCreator  Inputs=NumberofInputs
  Bus Creator1 : BusCreator  Inputs=2
  Bus Selector : BusSelector  OutputSignals=VehicleControlUnit,BUS.Driver and Enironment,BUS.DrivinCycle,BUS.Bus_Old  OutputAsBus=on
  BUS_OUT : Outport  VectorParamsAs1DForOutWhenUnconnected=off
  wires:
  Bus Creator1/1 -> Bus Selector/1
  BUS/1 -> Bus Creator1/1  "BUS"
  Bus Creator/1 -> Bus Creator1/2  "VehicleControlUnit"
  Bus Selector/1 -> BUS_OUT/1
  In1/1 -> Bus Creator/1  "TargetDriveTrq [Nm]"
  In2/1 -> Bus Creator/2  "TargetBrakeTrqFrontAxle [Nm]"
  In3/1 -> Bus Creator/3  "TargetBrakeTrqRearAxle [Nm]"

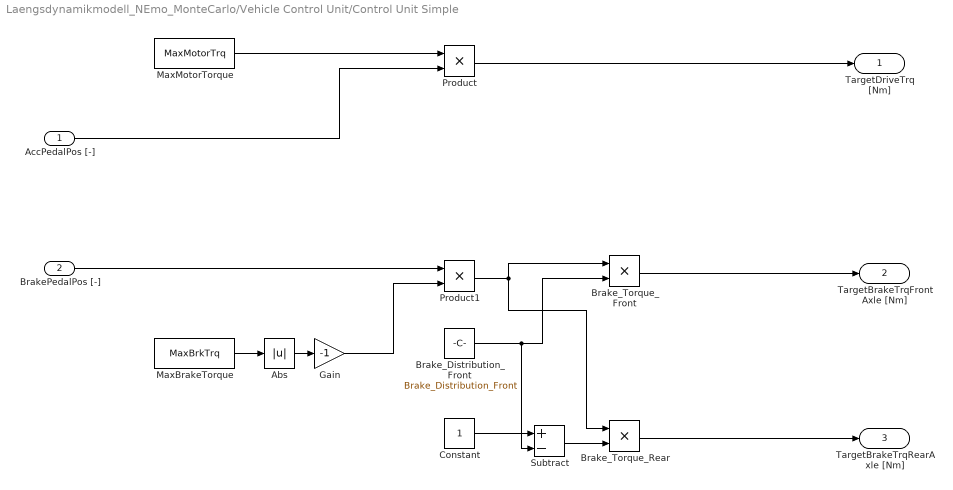
== system Laengsdynamikmodell_NEmo_MonteCarlo/Vehicle Control Unit/Control Unit Simple ==
  AccPedalPos [-] : Inport
  BrakePedalPos [-] : Inport  Port=2
  Abs : Abs
  Brake_Distribution_Front : Constant  Value=Brake_Distribution_Front
  Brake_Torque_Front : Product
  Brake_Torque_Rear : Product
  Constant : Constant
  Gain : Gain  Gain=-1
  MaxBrakeTorque : Constant  Value=MaxBrkTrq
  MaxMotorTorque : Constant  Value=MaxMotorTrq
  Product : Product
  Product1 : Product
  Subtract : Sum  Inputs=+-
  "TargetDriveTrq [Nm] " : Outport  VectorParamsAs1DForOutWhenUnconnected=off
  TargetBrakeTrqFrontAxle [Nm] : Outport  Port=2  VectorParamsAs1DForOutWhenUnconnected=off
  TargetBrakeTrqRearAxle [Nm] : Outport  Port=3  VectorParamsAs1DForOutWhenUnconnected=off
  wires:
  Gain/1 -> Product1/2
  Abs/1 -> Gain/1
  Product1/1 -> Brake_Torque_Front/1, Brake_Torque_Rear/1
  Brake_Distribution_Front/1 -> Brake_Torque_Front/2, Subtract/2
  MaxBrakeTorque/1 -> Abs/1
  Brake_Torque_Rear/1 -> TargetBrakeTrqRearAxle [Nm]/1
  AccPedalPos [-]/1 -> Product/2
  Constant/1 -> Subtract/1
  Subtract/1 -> Brake_Torque_Rear/2
  MaxMotorTorque/1 -> Product/1
  Brake_Torque_Front/1 -> TargetBrakeTrqFrontAxle [Nm]/1
  BrakePedalPos [-]/1 -> Product1/1
  Product/1 -> "TargetDriveTrq [Nm] "/1

== system Laengsdynamikmodell_NEmo_MonteCarlo/Powertrain/Electric Drive Tabled Consumption/LimitationElectricSystem ==
  OmegaMot [rad/s] : Inport
  MaxElectricPower [W] : Inport  Port=2
  MinElectricPower [W] : Inport  Port=3
  2-D Lookup Table1 : Lookup_n-D  BreakpointsForDimension1=OM_MotVector  BreakpointsForDimension2=PEl_MotVector  Table=OM_PEl_M_Map  UseLastTableValue=on  InternalRulePriority=Speed  RndMeth=Simplest  InputSameDT=on
  2-D Lookup Table3 : Lookup_n-D  BreakpointsForDimension1=OM_MotVector  BreakpointsForDimension2=PEl_MotVector  Table=OM_PEl_M_Map  UseLastTableValue=on  InternalRulePriority=Speed  RndMeth=Simplest  InputSameDT=on
  MaxTrqElectricLimit : Outport  VectorParamsAs1DForOutWhenUnconnected=off
  MinTrqElectricLimit : Outport  Port=2  VectorParamsAs1DForOutWhenUnconnected=off
  wires:
  2-D Lookup Table1/1 -> MaxTrqElectricLimit/1
  OmegaMot [rad/s]/1 -> 2-D Lookup Table1/1, 2-D Lookup Table3/1
  2-D Lookup Table3/1 -> MinTrqElectricLimit/1
  MinElectricPower [W]/1 -> 2-D Lookup Table3/2
  MaxElectricPower [W]/1 -> 2-D Lookup Table1/2

== system Laengsdynamikmodell_NEmo_MonteCarlo/Powertrain/Electric Drive Tabled Consumption/LimitationMechanicalSystem ==
  OmegaMot [rad/s] : Inport
  MaxTorqueLimitCurve : Lookup_n-D  NumberOfTableDimensions=1  BreakpointsForDimension1=OM_Full_Load  Table=M_Full_Load  InternalRulePriority=Speed  RndMeth=Simplest  InputSameDT=on
  MinTorqueLimitCurve : Lookup_n-D  NumberOfTableDimensions=1  BreakpointsForDimension1=OM_Min_Load  Table=M_Min_Load  InternalRulePriority=Speed  RndMeth=Simplest  InputSameDT=on
  MaxTrqMechanicalLimit : Outport  VectorParamsAs1DForOutWhenUnconnected=off
  MinTrqMechanicalLimit : Outport  Port=2  VectorParamsAs1DForOutWhenUnconnected=off
  wires:
  OmegaMot [rad/s]/1 -> MinTorqueLimitCurve/1, MaxTorqueLimitCurve/1
  MaxTorqueLimitCurve/1 -> MaxTrqMechanicalLimit/1
  MinTorqueLimitCurve/1 -> MinTrqMechanicalLimit/1
